simulink model "Nernst_RLS"  (R2015b)
settings: Solver=VariableStepAuto  StartTime=0.0  StopTime=7000  FixedStep=1/10  RelTol=1e-3
values from neighbouring files (symbols this model uses):
  cell_A123 =     [cells.mat]
  cell_sanyo =     [cells.mat]
undefined symbols (not defined in the file or in its folder): DiscIntNeverNeededParam
libraries: simulink x6, slident x2
settings Model: Creator=eprakE  LastModifiedBy=eprakE
settings DebuggingCC: InheritedTsInSrcMsg=none

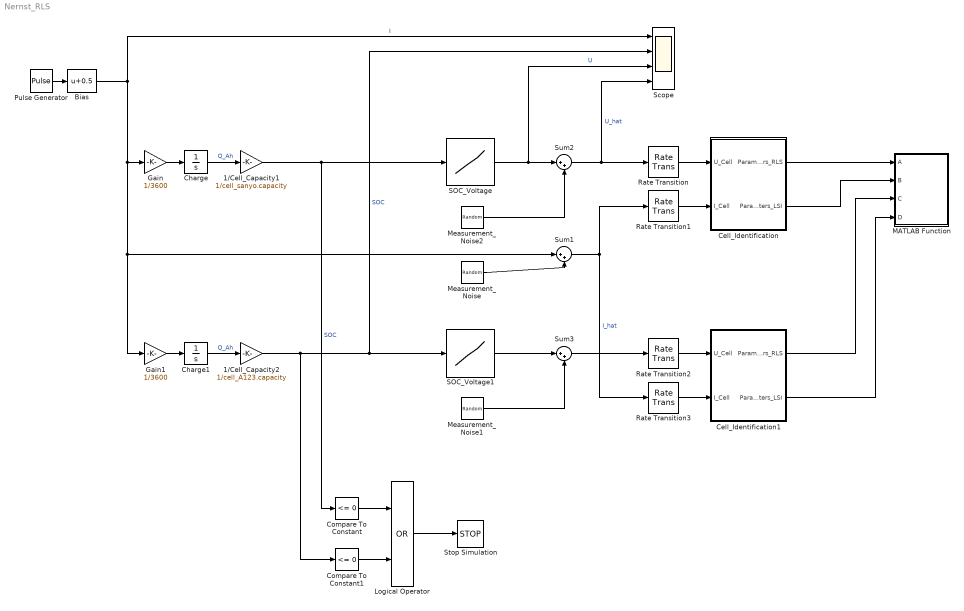
== system Nernst_RLS ==
  1/Cell_Capacity1 : Gain  Gain=1/cell_sanyo.capacity
  1/Cell_Capacity2 : Gain  Gain=1/cell_A123.capacity
  Bias : Bias  Bias=0.5
  Cell_Identification : Subsystem  TreatAsAtomicUnit=on  SystemSampleTime=1
  Cell_Identification1 : Subsystem  TreatAsAtomicUnit=on  SystemSampleTime=1
  Charge : Integrator  InitialCondition=2
  Charge1 : Integrator  InitialCondition=1
  Compare To Constant : simulink/Logic and Bit Operations/Compare To Constant  relop=<=  const=0  OutDataTypeStr=boolean
  Compare To Constant1 : simulink/Logic and Bit Operations/Compare To Constant  relop=<=  const=0  OutDataTypeStr=boolean
  Gain : Gain  Gain=1/3600
  Gain1 : Gain  Gain=1/3600
  Logical Operator : Logic  Operator=OR  AllPortsSameDT=off  OutDataTypeStr=boolean
  MATLAB Function : MATLAB Function  TreatAsAtomicUnit=on
  Measurement_Noise : RandomNumber  Variance=10e-3
  Measurement_Noise1 : RandomNumber  Variance=1e-6  Seed=2
  Measurement_Noise2 : RandomNumber  Variance=1e-6  Seed=1
  Pulse Generator : DiscretePulseGenerator  PulseType=Time based  Amplitude=-2  Period=10  PulseWidth=50
  Rate Transition{,1..3} (4 alike) : RateTransition
  SOC_Voltage : Lookup_n-D  NumberOfTableDimensions=1  BreakpointsForDimension1=cell_sanyo.soc  BeginIndexSearchUsingPreviousIndexResult=on  Table=cell_sanyo.voltage  InternalRulePriority=Speed  RndMeth=Simplest  InputSameDT=on
  SOC_Voltage1 : Lookup_n-D  NumberOfTableDimensions=1  BreakpointsForDimension1=cell_A123.soc  BeginIndexSearchUsingPreviousIndexResult=on  Table=cell_A123.voltage  InternalRulePriority=Speed  RndMeth=Simplest  InputSameDT=on
  Scope : Scope  NumInputPorts=4
  Stop Simulation : Stop
  Sum1 : Sum  Inputs=|++
  Sum2 : Sum  Inputs=|++
  Sum3 : Sum  Inputs=|++
  wires:
  Sum1/1 -> Rate Transition3/1, Rate Transition1/1  "I_hat"
  Measurement_Noise/1 -> Sum1/2
  Measurement_Noise2/1 -> Sum2/2
  Charge/1 -> 1/Cell_Capacity1/1  "Q_Ah"
  1/Cell_Capacity1/1 -> SOC_Voltage/1, Compare To Constant/1  "SOC"
  Pulse Generator/1 -> Bias/1
  SOC_Voltage/1 -> Scope/3, Sum2/1  "U"
  Sum2/1 -> Scope/4, Rate Transition/1  "U_hat"
  Bias/1 -> Scope/1, Gain/1, Gain1/1, Sum1/1  "I"
  Rate Transition/1 -> Cell_Identification/1(U_Cell)
  Rate Transition1/1 -> Cell_Identification/2(I_Cell)
  Gain/1 -> Charge/1
  Cell_Identification/1(Parameters_RLS) -> MATLAB Function/1(A)
  Rate Transition2/1 -> Cell_Identification1/1(U_Cell)
  Rate Transition3/1 -> Cell_Identification1/2(I_Cell)
  SOC_Voltage1/1 -> Sum3/1
  Sum3/1 -> Rate Transition2/1
  Measurement_Noise1/1 -> Sum3/2
  Charge1/1 -> 1/Cell_Capacity2/1  "Q_Ah"
  Gain1/1 -> Charge1/1
  1/Cell_Capacity2/1 -> Compare To Constant1/1, Scope/2, SOC_Voltage1/1  "SOC"
  Logical Operator/1 -> Stop Simulation/1
  Compare To Constant/1 -> Logical Operator/1
  Compare To Constant1/1 -> Logical Operator/2
  Cell_Identification1/1(Parameters_RLS) -> MATLAB Function/3(C)
  Cell_Identification/2(Parameters_LSI) -> MATLAB Function/2(B)
  Cell_Identification1/2(Parameters_LSI) -> MATLAB Function/4(D)

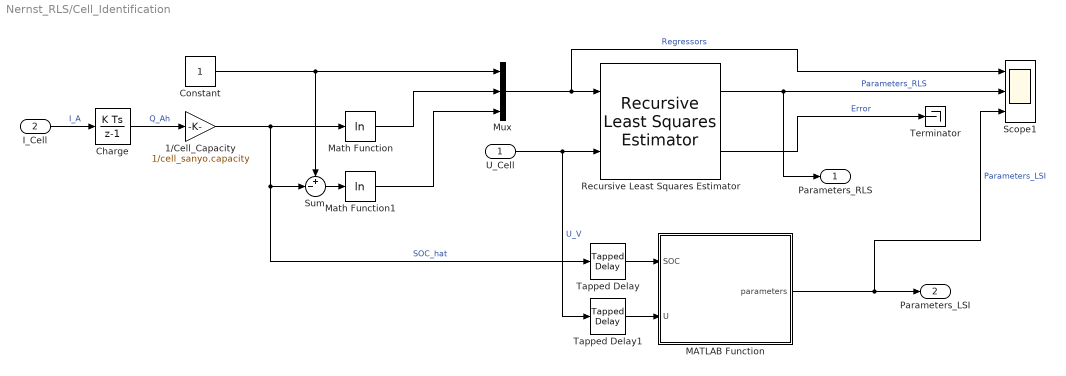
== system Nernst_RLS/Cell_Identification ==
  U_Cell : Inport
  I_Cell : Inport  Port=2
  1/Cell_Capacity : Gain  Gain=1/cell_sanyo.capacity
  Charge : DiscreteIntegrator  gainval=1/3600  InitialCondition=2  InitialConditionSetting=State (most efficient)  SampleTime=-1  ICPrevOutput=DiscIntNeverNeededParam  ICPrevScaledInput=DiscIntNeverNeededParam
  Constant : Constant
  MATLAB Function : MATLAB Function  TreatAsAtomicUnit=on
  Math Function : Math  Operator=log  SaturateOnIntegerOverflow=on
  Math Function1 : Math  Operator=log  SaturateOnIntegerOverflow=on
  Mux : Mux  Inputs=3
  Recursive Least Squares Estimator : slident/Estimators/Recursive Least Squares Estimator  InitialEstimateSource=Internal  InitialParameterData=[3 1 -1]  P0=eye(3)  EstimationMethod=Forgetting Factor  AdaptationParameter=0.9996  NormalizationBias=eps  OutputError=on  OutputP=off  AddEnablePort=off  Ts=-1
  Scope1 : Scope  NumInputPorts=3
  Sum : Sum  Inputs=+-|
  Tapped Delay : simulink/Discrete/Tapped Delay  vinit=0.0  samptime=-1  NumDelays=499  DelayOrder=Newest  includeCurrent=on
  Tapped Delay1 : simulink/Discrete/Tapped Delay  vinit=0.0  samptime=-1  NumDelays=499  DelayOrder=Newest  includeCurrent=on
  Terminator : Terminator
  Parameters_RLS : Outport
  Parameters_LSI : Outport  Port=2
  wires:
  Mux/1 -> Scope1/1, Recursive Least Squares Estimator/1  "Regressors"
  Recursive Least Squares Estimator/1 -> Parameters_RLS/1, Scope1/2  "Parameters_RLS"
  Recursive Least Squares Estimator/2 -> Terminator/1  "Error"
  U_Cell/1 -> Tapped Delay1/1, Recursive Least Squares Estimator/2  "U_V"
  Constant/1 -> Sum/1, Mux/1
  I_Cell/1 -> Charge/1  "I_A"
  Charge/1 -> 1/Cell_Capacity/1  "Q_Ah"
  1/Cell_Capacity/1 -> Tapped Delay/1, Sum/2, Math Function/1  "SOC_hat"
  Sum/1 -> Math Function1/1
  Math Function/1 -> Mux/2
  Math Function1/1 -> Mux/3
  MATLAB Function/1(parameters) -> Scope1/3, Parameters_LSI/1  "Parameters_LSI"
  Tapped Delay/1 -> MATLAB Function/1(SOC)
  Tapped Delay1/1 -> MATLAB Function/2(U)

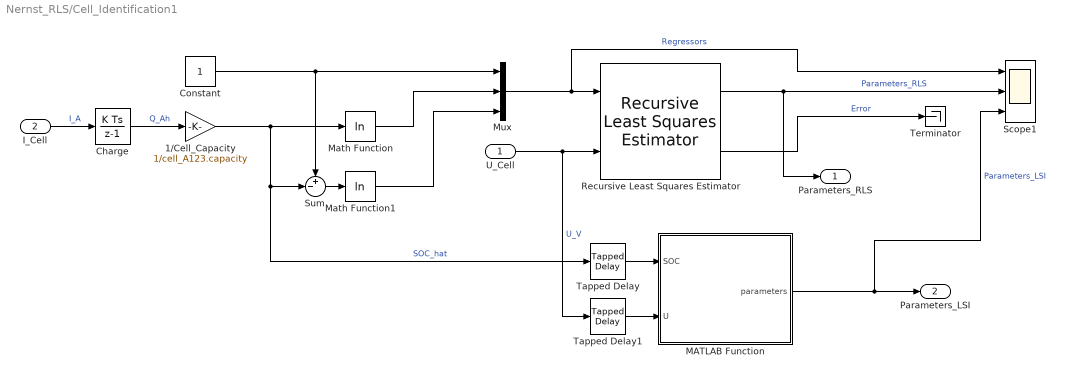
== system Nernst_RLS/Cell_Identification1 ==
  U_Cell : Inport
  I_Cell : Inport  Port=2
  1/Cell_Capacity : Gain  Gain=1/cell_A123.capacity
  Charge : DiscreteIntegrator  gainval=1/3600  InitialCondition=1  InitialConditionSetting=State (most efficient)  SampleTime=-1  ICPrevOutput=DiscIntNeverNeededParam  ICPrevScaledInput=DiscIntNeverNeededParam
  Constant : Constant
  MATLAB Function : MATLAB Function  TreatAsAtomicUnit=on
  Math Function : Math  Operator=log  SaturateOnIntegerOverflow=on
  Math Function1 : Math  Operator=log  SaturateOnIntegerOverflow=on
  Mux : Mux  Inputs=3
  Recursive Least Squares Estimator : slident/Estimators/Recursive Least Squares Estimator  InitialEstimateSource=Internal  InitialParameterData=[3 1 -1]  P0=eye(3)  EstimationMethod=Forgetting Factor  AdaptationParameter=0.9996  NormalizationBias=eps  OutputError=on  OutputP=off  AddEnablePort=off  Ts=-1
  Scope1 : Scope  NumInputPorts=3
  Sum : Sum  Inputs=+-|
  Tapped Delay : simulink/Discrete/Tapped Delay  vinit=0.0  samptime=-1  NumDelays=499  DelayOrder=Newest  includeCurrent=on
  Tapped Delay1 : simulink/Discrete/Tapped Delay  vinit=0.0  samptime=-1  NumDelays=499  DelayOrder=Newest  includeCurrent=on
  Terminator : Terminator
  Parameters_RLS : Outport
  Parameters_LSI : Outport  Port=2
  wires:
  Tapped Delay1/1 -> MATLAB Function/2(U)
  Tapped Delay/1 -> MATLAB Function/1(SOC)
  MATLAB Function/1(parameters) -> Parameters_LSI/1, Scope1/3  "Parameters_LSI"
  Math Function1/1 -> Mux/3
  Math Function/1 -> Mux/2
  Sum/1 -> Math Function1/1
  1/Cell_Capacity/1 -> Math Function/1, Sum/2, Tapped Delay/1  "SOC_hat"
  Charge/1 -> 1/Cell_Capacity/1  "Q_Ah"
  I_Cell/1 -> Charge/1  "I_A"
  Constant/1 -> Mux/1, Sum/1
  U_Cell/1 -> Recursive Least Squares Estimator/2, Tapped Delay1/1  "U_V"
  Recursive Least Squares Estimator/2 -> Terminator/1  "Error"
  Recursive Least Squares Estimator/1 -> Scope1/2, Parameters_RLS/1  "Parameters_RLS"
  Mux/1 -> Recursive Least Squares Estimator/1, Scope1/1  "Regressors"

== matlab function Nernst_RLS/Cell_Identification/MATLAB Function ==
  data: SOC input; parameters output; U input
function parameters = fcn(SOC, U)

C = [ones(length(U), 1), log(SOC), log(1 - SOC)];
A = [-1,  0, 0;
      0, -1, 0;
      0,  0, 1];
b = [-3,  0, 0];

parameters = zeros(3, 1);

coder.extrinsic('lsqlin');
parameters = lsqlin(C, U, A, b);

== matlab function Nernst_RLS/MATLAB Function ==
  data: A input; B input; C input; D input
function fcn(A, B, C, D)
%#codegen

SOC = linspace(1e-3, 0.999);
U = zeros(4, 100);
U(1, :) = A(1) + A(2)*log(SOC) + A(3)*log(1 - SOC);
U(2, :) = B(1) + B(2)*log(SOC) + B(3)*log(1 - SOC);
U(3, :) = C(1) + C(2)*log(SOC) + C(3)*log(1 - SOC);
U(4, :) = D(1) + D(2)*log(SOC) + D(3)*log(1 - SOC);

coder.extrinsic('legend');

subplot(1, 2, 1);
plot(SOC, U(1, :));
hold on;
plot(SOC, U(2, :));
hold off;
grid on;
title('Sanyo');
xlabel('SOC');
ylabel('U');
xlim([0 1]);
ylim([2 4.5]);
legend('RLS', 'LSI');

subplot(1, 2, 2);
plot(SOC, U(3, :));
hold on;
plot(SOC, U(4, :));
hold off;
grid on;
title('A123');
xlabel('SOC');
ylabel('U');
xlim([0 1]);
ylim([2 4.5]);
legend('RLS', 'LSI');

== matlab function Nernst_RLS/Cell_Identification1/MATLAB Function ==
  data: SOC input; parameters output; U input
function parameters = fcn(SOC, U)

C = [ones(length(U), 1), log(SOC), log(1 - SOC)];
A = [-1,  0, 0;
      0, -1, 0;
      0,  0, 1];
b = [-3,  0, 0];

parameters = zeros(3, 1);

coder.extrinsic('lsqlin');
parameters = lsqlin(C, U, A, b);
